simulink model "Problem3"  (R2020a)
settings: Solver=VariableStepAuto  StartTime=0.0  StopTime=10.0  RelTol=1e-3
model workspace (MAT data in the model file):
  A = 0.5792
  B = -0.5792
  C = 0.158
settings Model: Creator=sreeram  LastModifiedBy=sreeram

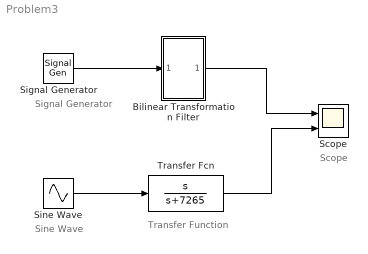
== system Problem3 ==
  note: Scope
  note: Transfer Function
  note: Sine Wave
  note: Signal
      | Generator
  Bilinear Transformation Filter : Subsystem
  Scope : Scope  NumInputPorts=2
  Signal Generator : SignalGenerator  Units=rad/sec
  Sine Wave : Sin  Frequency=3455.75  SampleTime=0
  Transfer Fcn : TransferFcn  Numerator=[1 0]  Denominator=[1 7265]
  wires:
  Sine Wave/1 -> Transfer Fcn/1
  Transfer Fcn/1 -> Scope/2
  Signal Generator/1 -> Bilinear Transformation Filter/1(In1)
  Bilinear Transformation Filter/1(Out1) -> Scope/1

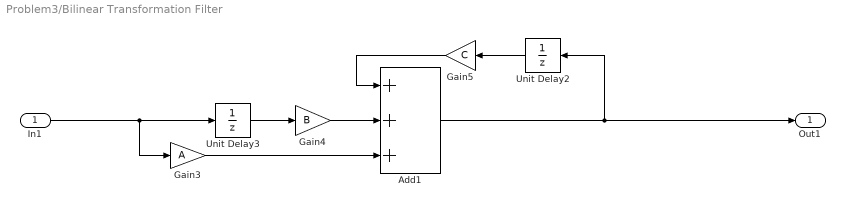
== system Problem3/Bilinear Transformation Filter ==
  In1 : Inport
  Add1 : Sum  Inputs=+++
  Gain3 : Gain  Gain=A
  Gain4 : Gain  Gain=B
  Gain5 : Gain  Gain=C
  Unit Delay2 : UnitDelay  SampleTime=-1  HasFrameUpgradeWarning=on
  Unit Delay3 : UnitDelay  SampleTime=-1  HasFrameUpgradeWarning=on
  Out1 : Outport
  wires:
  Unit Delay3/1 -> Gain4/1
  Gain5/1 -> Add1/1
  Add1/1 -> Out1/1, Unit Delay2/1
  Gain3/1 -> Add1/3
  Gain4/1 -> Add1/2
  Unit Delay2/1 -> Gain5/1
  In1/1 -> Gain3/1, Unit Delay3/1
